simulink model "Par6"  (R2018a)
settings: Solver=FixedStepAuto  StartTime=0.0  StopTime=10  FixedStep=0.1  RelTol=1e-3
settings Model: Creator=wangluo  LastModifiedBy=wangluo

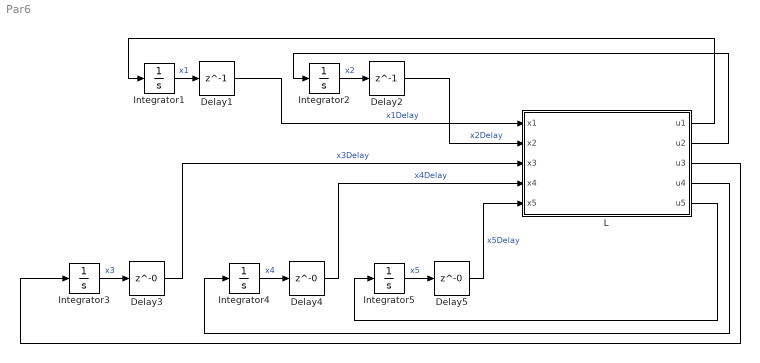
== system Par6 ==
  Delay1 : Delay  DelayLength=1  InitialCondition=0
  Delay2 : Delay  DelayLength=1  InitialCondition=0
  Delay3 : Delay  DelayLength=0  InitialCondition=0
  Delay4 : Delay  DelayLength=0  InitialCondition=0
  Delay5 : Delay  DelayLength=0  InitialCondition=0
  Integrator1 : Integrator  InitialCondition=-4
  Integrator2 : Integrator  InitialCondition=5
  Integrator3 : Integrator  InitialCondition=-6
  Integrator4 : Integrator  InitialCondition=7
  Integrator5 : Integrator  InitialCondition=-8
  L : Subsystem
  wires:
  Integrator1/1 -> Delay1/1  "x1"
  Integrator2/1 -> Delay2/1  "x2"
  Integrator3/1 -> Delay3/1  "x3"
  L/2(u2) -> Integrator2/1
  L/1(u1) -> Integrator1/1
  L/3(u3) -> Integrator3/1
  L/4(u4) -> Integrator4/1
  L/5(u5) -> Integrator5/1
  Delay4/1 -> L/4(x4)  "x4Delay"
  Delay3/1 -> L/3(x3)  "x3Delay"
  Delay5/1 -> L/5(x5)  "x5Delay"
  Delay1/1 -> L/1(x1)  "x1Delay"
  Delay2/1 -> L/2(x2)  "x2Delay"
  Integrator4/1 -> Delay4/1  "x4"
  Integrator5/1 -> Delay5/1  "x5"

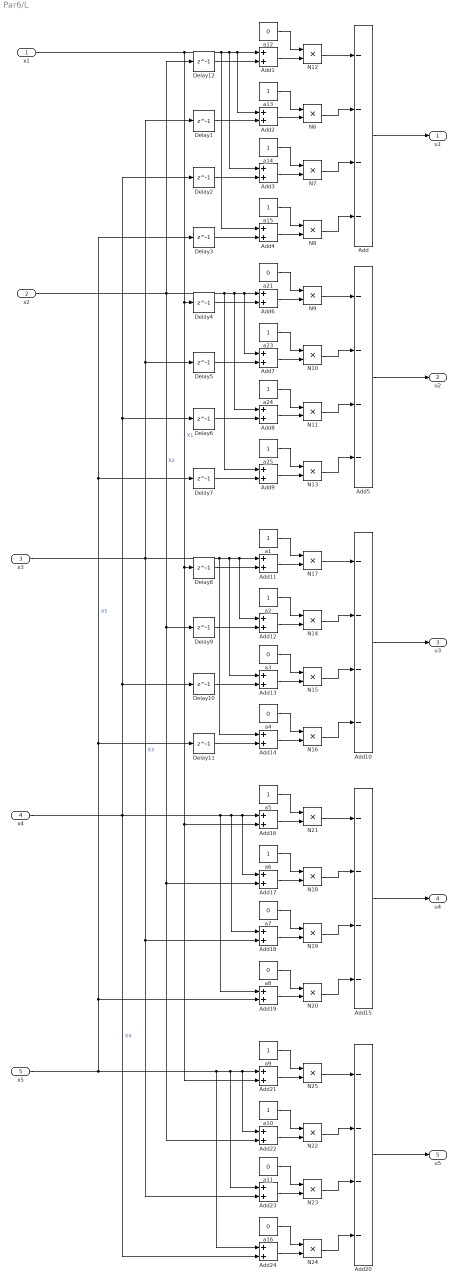
== system Par6/L ==
  x1 : Inport
  x2 : Inport  Port=2
  x3 : Inport  Port=3
  x4 : Inport  Port=4
  x5 : Inport  Port=5
  Add{,5,10,15,20} (5 alike) : Sum  Inputs=----
  Add{1..4,6..9,11..14,16..19,21..24} (20 alike) : Sum
  Delay{1..12} (12 alike) : Delay  DelayLength=1  InitialCondition=0
  N{6..25} (20 alike) : Product
  a{1..2,5..6,9..10,13..15,23..25} (12 alike) : Constant
  a{3..4,7..8,11..12,16,21} (8 alike) : Constant  Value=0
  u1 : Outport
  u2 : Outport  Port=2
  u3 : Outport  Port=3
  u4 : Outport  Port=4
  u5 : Outport  Port=5
  wires:
  a12/1 -> N12/1
  N12/1 -> Add/1
  Add/1 -> u1/1
  x1/1 -> Delay4/1, Add16/2, Add21/2, Delay8/1, Add4/1, Add3/1, Add1/1, Add2/1  "X1"
  x2/1 -> Add9/1, Add8/1, Add7/1, Add6/1, Add22/2, Add17/2, Delay9/1, Delay12/1  "X2"
  Add1/1 -> N12/2
  Add2/1 -> N6/2
  a13/1 -> N6/1
  N6/1 -> Add/2
  Add3/1 -> N7/2
  a14/1 -> N7/1
  N7/1 -> Add/3
  Add4/1 -> N8/2
  a15/1 -> N8/1
  N8/1 -> Add/4
  x3/1 -> Add23/2, Add18/2, Delay1/1, Delay5/1, Add14/1, Add13/1, Add12/1, Add11/1  "X3"
  x4/1 -> Add24/2, Add19/1, Add18/1, Add17/1, Add16/1, Delay10/1, Delay2/1, Delay6/1  "X4"
  x5/1 -> Delay3/1, Delay7/1, Delay11/1, Add19/2, Add23/1, Add22/1, Add21/1, Add24/1  "X5"
  N10/1 -> Add5/2
  Add6/1 -> N9/2
  N9/1 -> Add5/1
  Add5/1 -> u2/1
  Add7/1 -> N10/2
  Add9/1 -> N13/2
  a21/1 -> N9/1
  N11/1 -> Add5/3
  N13/1 -> Add5/4
  a23/1 -> N10/1
  a25/1 -> N13/1
  Add8/1 -> N11/2
  a24/1 -> N11/1
  Add12/1 -> N14/2
  N15/1 -> Add10/3
  Add11/1 -> N17/2
  a4/1 -> N16/1
  a3/1 -> N15/1
  a2/1 -> N14/1
  Add13/1 -> N15/2
  N14/1 -> Add10/2
  Add14/1 -> N16/2
  N16/1 -> Add10/4
  a1/1 -> N17/1
  N17/1 -> Add10/1
  Add10/1 -> u3/1
  Add17/1 -> N18/2
  N19/1 -> Add15/3
  a7/1 -> N19/1
  Add19/1 -> N20/2
  a6/1 -> N18/1
  Add16/1 -> N21/2
  N18/1 -> Add15/2
  Add18/1 -> N19/2
  N20/1 -> Add15/4
  a8/1 -> N20/1
  a5/1 -> N21/1
  N21/1 -> Add15/1
  Add23/1 -> N23/2
  N22/1 -> Add20/2
  a16/1 -> N24/1
  N24/1 -> Add20/4
  Add22/1 -> N22/2
  a11/1 -> N23/1
  a10/1 -> N22/1
  N25/1 -> Add20/1
  a9/1 -> N25/1
  Add21/1 -> N25/2
  Add24/1 -> N24/2
  N23/1 -> Add20/3
  Add15/1 -> u4/1
  Add20/1 -> u5/1
  Delay12/1 -> Add1/2
  Delay1/1 -> Add2/2
  Delay2/1 -> Add3/2
  Delay3/1 -> Add4/2
  Delay4/1 -> Add6/2
  Delay5/1 -> Add7/2
  Delay6/1 -> Add8/2
  Delay7/1 -> Add9/2
  Delay8/1 -> Add11/2
  Delay9/1 -> Add12/2
  Delay10/1 -> Add13/2
  Delay11/1 -> Add14/2
